simulink model "stridac_1f"  (Simulink 8.0)
settings: Solver=ode1  StartTime=0.0  StopTime=1  FixedStep=1e-5  MaxStep=1e-5  RelTol=1e-3
undefined symbols (not defined in the file): plecsedit
libraries: simulink x1
settings Model: Creator=dragounj  LastModifiedBy=Kasi
settings DataIOCC: SignalLoggingSaveFormat=ModelDataLogs
settings DebuggingCC: FcnCallInpInsideContextMsg=UseLocalSettings
settings GRTTargetCC: CombineOutputUpdateFcns=off  GRTInterface=on

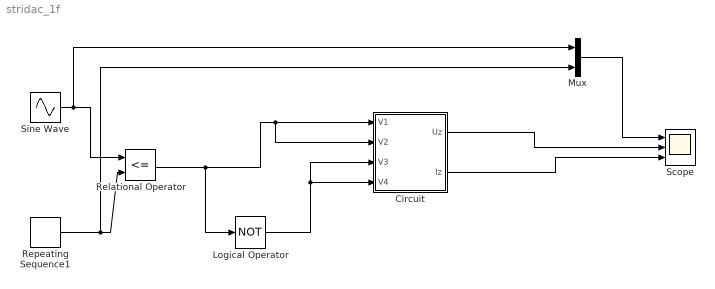
== system stridac_1f ==
  Circuit : Subsystem  LoadFcn=plecsedit('sl', 200);  InitFcn=plecsedit('sl', 214);  StartFcn=plecsedit('sl', 208);  StopFcn=plecsedit('sl', 209);  mask(PlecsCircuit){}
      mask init:
      | % PLACE CUSTOM INITIALIZATIONS ABOVE
      | % DO NOT REMOVE
      | plecsedit('sl', 215);
      | % DO NOT REMOVE
      settings: CopyFcn=plecsedit('sl', 203);  DeleteFcn=plecsedit('sl', 205);  UndoDeleteFcn=plecsedit('sl', 206);  PreSaveFcn=plecsedit('sl', 211);  PostSaveFcn=plecsedit('sl', 201);  NameChangeFcn=plecsedit('sl', 210);  DestroyFcn=plecsedit('sl', 207);  PreCopyFcn=plecsedit('sl', 216);  OpenFcn=plecsedit('sl', 202);  ErrorFcn=plerrorfcn
      mask Display: disp('PLECS\nCircuit')
  Logical Operator : Logic  Operator=NOT  AllPortsSameDT=off  OutDataTypeStr=boolean
  Mux : Mux  Inputs=2
  Relational Operator : RelationalOperator  Operator=<=  OutDataTypeStr=boolean
  Repeating Sequence1 : simulink/Sources/Repeating Sequence  rep_seq_t=[0 0.5 1]/500  rep_seq_y=[-1 1 -1]
  Scope : Scope  NumInputPorts=3
      settings: YMin=-5~-5~-5  YMax=5~5~5
  Sine Wave : Sin  Frequency=50  SampleTime=0
  wires:
  Sine Wave/1 -> Mux/1, Relational Operator/1
  Repeating Sequence1/1 -> Mux/2, Relational Operator/2
  Relational Operator/1 -> Circuit/1(V1), Circuit/2(V2), Logical Operator/1
  Logical Operator/1 -> Circuit/3(V3), Circuit/4(V4)
  Mux/1 -> Scope/1
  Circuit/1(Uz) -> Scope/2
  Circuit/2(Iz) -> Scope/3

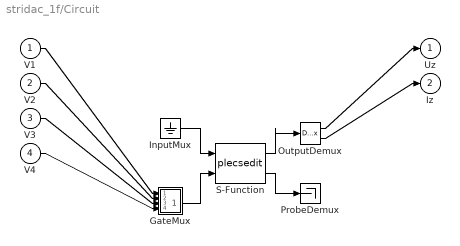
== system stridac_1f/Circuit ==
  V1 : Inport  PortDimensions=1
  V2 : Inport  Port=2  PortDimensions=1
  V3 : Inport  Port=3  PortDimensions=1
  V4 : Inport  Port=4  PortDimensions=1
  " GateMux " : Subsystem
      mask Display: disp('Mux')
  " InputMux " : Ground
  " OutputDemux " : Demux  Outputs=[ 1 1 ]
  " ProbeDemux " : Terminator
  " S-Function " : S-Function  FunctionName=plecsedit  EnableBusSupport=off
  Uz : Outport  PortDimensions=1
  Iz : Outport  Port=2  PortDimensions=1
  wires:
  " S-Function "/1 -> " OutputDemux "/1
  " InputMux "/1 -> " S-Function "/1
  " GateMux "/1(Out) -> " S-Function "/2
  " S-Function "/2 -> " ProbeDemux "/1
  V1/1 -> " GateMux "/1(In1)
  V2/1 -> " GateMux "/2(In2)
  V3/1 -> " GateMux "/3(In3)
  V4/1 -> " GateMux "/4(In4)
  " OutputDemux "/1 -> Uz/1
  " OutputDemux "/2 -> Iz/1

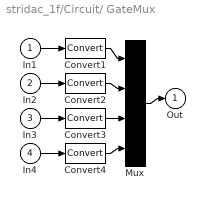
== system stridac_1f/Circuit/ GateMux  ==
  In1 : Inport
  In2 : Inport  Port=2
  In3 : Inport  Port=3
  In4 : Inport  Port=4
  Convert{1..4} (4 alike) : DataTypeConversion  SaturateOnIntegerOverflow=on  RndMeth=Zero
  Mux : Mux  Inputs=[ 1 1 1 1 ]
  Out : Outport
  wires:
  Mux/1 -> Out/1
  In1/1 -> Convert1/1
  In2/1 -> Convert2/1
  In3/1 -> Convert3/1
  In4/1 -> Convert4/1
  Convert1/1 -> Mux/1
  Convert2/1 -> Mux/2
  Convert3/1 -> Mux/3
  Convert4/1 -> Mux/4
